simulink model "Gatepluse_SCBI"  (R2018a)
settings: Solver=VariableStepAuto  StartTime=0.0  StopTime=0.02  RelTol=1e-3
libraries: simulink x4, powerlib x1
settings Model: Creator=asus  LastModifiedBy=asus

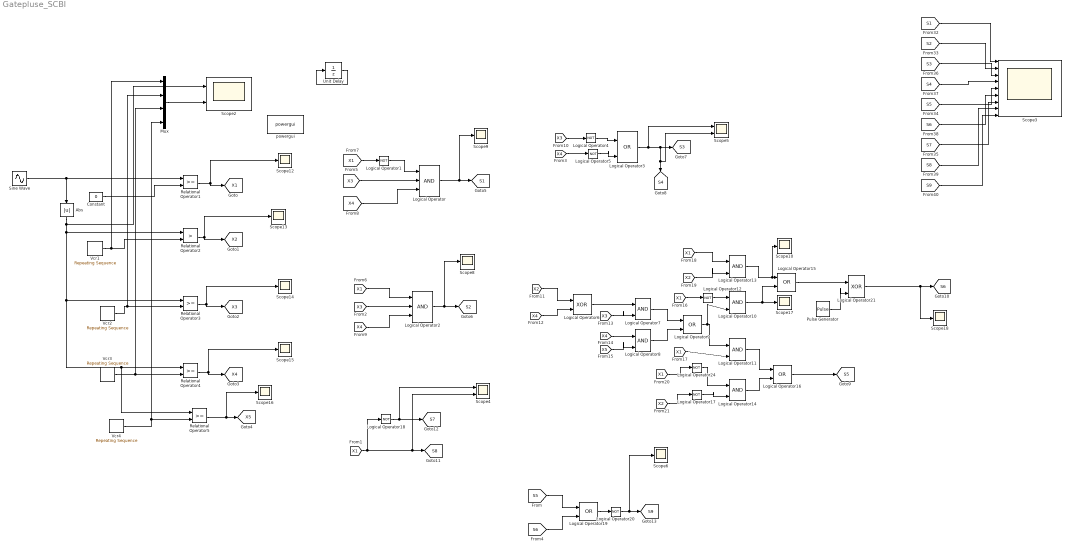
== system Gatepluse_SCBI ==
  Abs : Abs
  Constant : Constant  Value=0
  Logical Operator : Logic  Inputs=3  IconShape=distinctive  AllPortsSameDT=off  OutDataTypeStr=boolean
  Logical Operator{1,4..5,12,17..18,20,24} (8 alike) : Logic  Operator=NOT  Inputs=3  IconShape=distinctive  AllPortsSameDT=off  OutDataTypeStr=boolean
  Logical Operator{7..8,10..11,13..14} (6 alike) : Logic  IconShape=distinctive  AllPortsSameDT=off  OutDataTypeStr=boolean
  Logical Operator{3,9,15..16,19} (5 alike) : Logic  Operator=OR  IconShape=distinctive  AllPortsSameDT=off  OutDataTypeStr=boolean
  Logical Operator2 : Logic  Inputs=3  IconShape=distinctive  AllPortsSameDT=off  OutDataTypeStr=boolean
  Logical Operator21 : Logic  Operator=XOR  IconShape=distinctive  AllPortsSameDT=off  OutDataTypeStr=boolean
  Logical Operator6 : Logic  Operator=XOR  IconShape=distinctive  AllPortsSameDT=off  OutDataTypeStr=boolean
  Mux : Mux
  Pulse Generator : DiscretePulseGenerator  PulseType=Time based  Period=0.02  PulseWidth=50
  Relational Operator{1,3..5} (4 alike) : RelationalOperator  OutDataTypeStr=boolean  RndMeth=Simplest
  Relational Operator2 : RelationalOperator  Operator=>  OutDataTypeStr=boolean  RndMeth=Simplest
  Scope{6,8..10,12..18} (11 alike) : Scope
  Scope2 : Scope  NumInputPorts=2
  Scope3 : Scope  NumInputPorts=9
  Scope4 : Scope  NumInputPorts=2
  Scope5 : Scope  NumInputPorts=2
  Sine Wave : Sin  Amplitude=3.9  Frequency=2*pi*50  SampleTime=1e-6
  Unit Delay : UnitDelay  SampleTime=-1
  Vcr1 : simulink/Sources/Repeating Sequence  rep_seq_t=[0 0.0002 0.0004]  rep_seq_y=[0 1 0]
  Vcr2 : simulink/Sources/Repeating Sequence  rep_seq_t=[0 0.0002 0.0004]  rep_seq_y=[1 2 1]
  Vcr3 : simulink/Sources/Repeating Sequence  rep_seq_t=[0 0.0002 0.0004]  rep_seq_y=[2 3 2]
  Vcr4 : simulink/Sources/Repeating Sequence  rep_seq_t=[0 0.0002 0.0004]  rep_seq_y=[3 4 3]
  powergui : powerlib/powergui  Priority=1  SimulationMode=Continuous  SampleTime=50e-6  frequency=60  Iterations=50  frequencyindice=0  Pbase=100e6  ErrMax=1e-4  UnitsV=kV  UnitsW=MW  buscounter=0  FunctionMessages=off  echomessages=off  EnableUseOfTLC=off  CurrentSourceSwitches=off  DisableSnubberDevices=off  DisableRonSwitches=off  DisableVfSwitches=off  DisplayEquations=off  SolverType=Tustin/Backward Euler (TBE)  Interpol=off  ExternalGateDelay=off  methode=off  Ts=100  x0status=blocks  SPID=on  SwTol=0  HookPort=off  RestoreLinks=warning  ResistiveCurrentMeasurement=off  Frange=[0:2:500]  Ylog=off  Xlog=on  ShowGrid=off  save=off  variable=ZData  structure=0  ZoomFFT=off  StartTime=0.0  cycles=1  DisplayStyle=1  fundamental=60  FreqAxis=off  MaxFrequency=1000  frequencyindicesteady=1  RmsSteady=1  display=off
  tag scope: S1=global, S2=global, S3=global, S4=global, S5=global, S6=global, S7=global, S8=global, S9=global, X1=global, X2=global, X3=global, X4=global, X5=global
  wires:
  [S6] -> Scope3/6
  Constant/1 -> Relational Operator1/2
  Unit Delay/1 -> Unit Delay/1
  [S4] -> Scope3/4
  [S3] -> Scope3/3
  Relational Operator5/1 -> [X5], Scope16/1
  [S7] -> Scope3/7
  Abs/1 -> Scope2/1, Relational Operator2/1, Relational Operator3/1, Relational Operator4/1, Relational Operator5/1
  [S8] -> Scope3/8
  [S9] -> Scope3/9
  Relational Operator1/1 -> [X1], Scope12/1
  Vcr1/1 -> Mux/1, Relational Operator2/2
  Relational Operator4/1 -> [X4], Scope15/1
  [S1] -> Scope3/1
  Vcr4/1 -> Mux/4, Relational Operator5/2
  [S2] -> Scope3/2
  Relational Operator3/1 -> [X3], Scope14/1
  Sine Wave/1 -> Abs/1, Relational Operator1/1
  Vcr3/1 -> Mux/3, Relational Operator4/2
  [S5] -> Scope3/5
  Relational Operator2/1 -> [X2], Scope13/1
  Vcr2/1 -> Mux/2, Relational Operator3/2
  Mux/1 -> Scope2/2
  [X1] -> Logical Operator12/1
  [X2] -> Logical Operator17/1
  [S6] -> Logical Operator19/2
  Logical Operator9/1 -> Logical Operator11/1, Logical Operator10/2
  Logical Operator6/1 -> Logical Operator7/1
  [X1] -> Logical Operator24/1
  [X4] -> Logical Operator5/1
  Logical Operator5/1 -> Logical Operator3/2
  [X3] -> Logical Operator2/2
  [X1] -> Logical Operator2/1
  [S5] -> Logical Operator19/1
  [X4] -> Logical Operator8/1
  [X4] -> Logical Operator/3
  [X4] -> Logical Operator2/3
  [X1] -> Logical Operator1/1
  [X3] -> Logical Operator/2
  Logical Operator10/1 -> Logical Operator15/2, Scope17/1
  Logical Operator14/1 -> Logical Operator16/2
  Logical Operator1/1 -> Logical Operator/1
  [X3] -> Logical Operator4/1
  Logical Operator12/1 -> Logical Operator10/1
  [X3] -> Logical Operator7/2
  Logical Operator4/1 -> Logical Operator3/1
  Logical Operator7/1 -> Logical Operator9/1
  Logical Operator11/1 -> Logical Operator16/1
  Logical Operator18/1 -> Scope4/1, [S7]
  Logical Operator8/1 -> Logical Operator9/2
  [X1] -> Logical Operator11/2
  Logical Operator13/1 -> Logical Operator15/1, Scope10/1
  Logical Operator17/1 -> Logical Operator14/2
  [X1] -> Logical Operator13/1
  Logical Operator2/1 -> Scope8/1, [S2]
  Logical Operator/1 -> Scope9/1, [S1]
  [X1] -> Logical Operator18/1, Scope4/2, [S8]
  [X2] -> Logical Operator13/2
  [X5] -> Logical Operator8/2
  Logical Operator19/1 -> Logical Operator20/1
  Logical Operator3/1 -> Scope5/1, Scope5/2, [S4], [S3]
  Logical Operator15/1 -> Logical Operator21/1
  [X2] -> Logical Operator6/1
  [X4] -> Logical Operator6/2
  Pulse Generator/1 -> Logical Operator21/2
  Logical Operator21/1 -> Scope18/1, [S6]
  Logical Operator16/1 -> [S5]
  Logical Operator24/1 -> Logical Operator14/1
  Logical Operator20/1 -> Scope6/1, [S9]
